simulink model "ESO_test"  (Simulink 8.8)
settings: Solver=ode45  StartTime=0.0  StopTime=10.0  RelTol=1e-3  EnableMultiTasking=on
values from neighbouring files (symbols this model uses):
  A = [-351.120003184 -5361.83522933 0 0 0 0 0 0 0 0 0 0 ... (196 elements, 14x14)]    [identified_modal.mat]    (also in identified_modal_250.mat = [-10.7295401852 -1238.51536589 0 0 0 0 1238.51536589 -10.729)
  Am = A    [ESO_performance_test.m]
  B = [573.623221602 72.4542684161 -691.638848987 228.937697811 -252.989182838 -22.7617436487 170.002545784 4.18017568557 -18.4488355601 113.905004057 -95.0717241213 -56.2996980805 ... (42 elements, 14x3)]    [identified_modal.mat]    (also in identified_modal_250.mat = [-1.29092394555 -1.97797965398 -0.850667801822 1.31545698651)
  Bm = B    [ESO_performance_test.m]
  C = [0.627446579032 0.0119792109415 0.587375916328 0.0249330272657 -0.39941806915 -0.0483765376125 0.228423611726 0.0697233755056 0.0235364777295 -0.0130974661322 0.147269800576 0.0117524583717 ... (28 elements, 2x14)]    [identified_modal.mat]    (also in identified_modal_250.mat = [-2.98376370972  6.90606082788  -5.3698593094  -1.7527268949)
  Cm = C    [ESO_performance_test.m]
  Cw = zeros(n_w,n_xw)    [ESO_design.m]    (also in ESO_performance_test.m)
  D = D(:,1:3)    [ESO_performance_test.m]    (also in identified_modal.mat = [-0.0335072369376  0.101109733478  0.0863325632373  -0.01405; identified_modal_250.mat = [-2.22661181806e-05  0.0283763020492  -0.000188131534199  0.)
  Dm = D    [ESO_performance_test.m]
  E = zeros(n_xw,n_h)    [ESO_design.m]    (also in ESO_performance_test.m)
  H = [33.6937621374 18.4906854499 -113.318027588 5.64627813379 9.51722897194 3.09854032404 -14.991856853 99.088587685 -7.37918928848 3.49318728719 21.2561682387 -20.6265244709 ... (14 elements, 14x1)]    [identified_modal.mat]    (also in identified_modal_250.mat = [0.0764124681014 0.0372004138976 0.178660840601 0.2484513591)
  Hm = H    [ESO_performance_test.m]
  L1 = L(1:n_x,:)    [ESO_performance_test.m]
  L2 = L(n_x+1:n_x+n_xw,:)    [ESO_performance_test.m]
  S = blkdiag(S,zeros(1,1))    [ESO_design.m]    (also in ESO_performance_test.m)
settings Model: Creator=Mehran  LastModifiedBy=ABLAH
settings OptimizationCC: ExpressionDepthLimit=2147483647
settings DebuggingCC: SolverPrmCheckMsg=warning

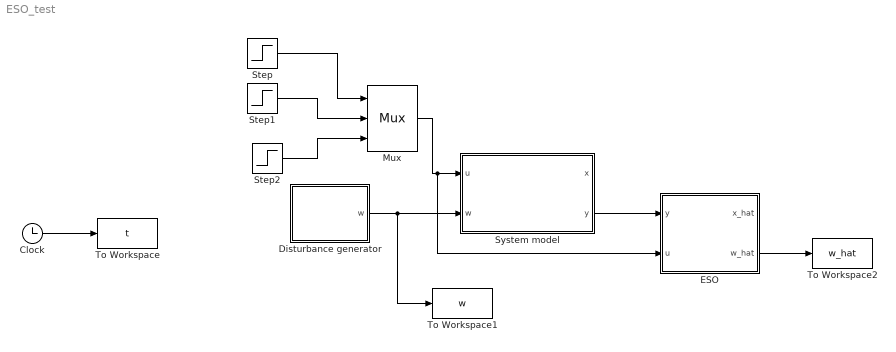
== system ESO_test ==
  Clock : Clock
  Disturbance generator : Subsystem
  ESO : Subsystem
  Mux : Mux  Inputs=3
  Step : Step  Time=0  After=0  SampleTime=0
  Step1 : Step  Time=0  After=0  SampleTime=0
  Step2 : Step  Time=0  After=0  SampleTime=0
  System model : Subsystem
  To Workspace : ToWorkspace  VariableName=t  SampleTime=-1
  To Workspace1 : ToWorkspace  VariableName=w  SampleTime=-1
  To Workspace2 : ToWorkspace  VariableName=w_hat  SampleTime=-1
  wires:
  Disturbance generator/1(w) -> System model/2(w), To Workspace1/1
  System model/2(y) -> ESO/1(y)
  Mux/1 -> System model/1(u), ESO/2(u)
  Step/1 -> Mux/1
  Step1/1 -> Mux/2
  Step2/1 -> Mux/3
  Clock/1 -> To Workspace/1
  ESO/2(w_hat) -> To Workspace2/1

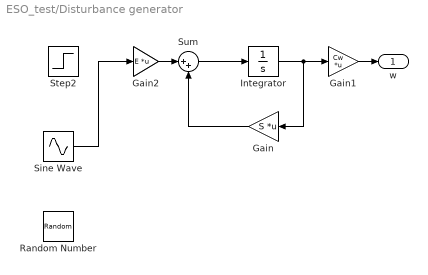
== system ESO_test/Disturbance generator ==
  Gain : Gain  Gain=S  Multiplication=Matrix(K*u)
  Gain1 : Gain  Gain=Cw  Multiplication=Matrix(K*u)
  Gain2 : Gain  Gain=E  Multiplication=Matrix(K*u)
  Integrator : Integrator  InitialCondition=0.1*[ones(12,1);0]
  Random Number : RandomNumber  SampleTime=0.1
  Sine Wave : Sin  Amplitude=3  Frequency=13.8  SampleTime=0
  Step2 : Step  Time=0  After=0  SampleTime=0
  Sum : Sum  Inputs=|++
  w : Outport
  wires:
  Integrator/1 -> Gain/1, Gain1/1
  Gain/1 -> Sum/2
  Sum/1 -> Integrator/1
  Gain1/1 -> w/1
  Gain2/1 -> Sum/1
  Sine Wave/1 -> Gain2/1

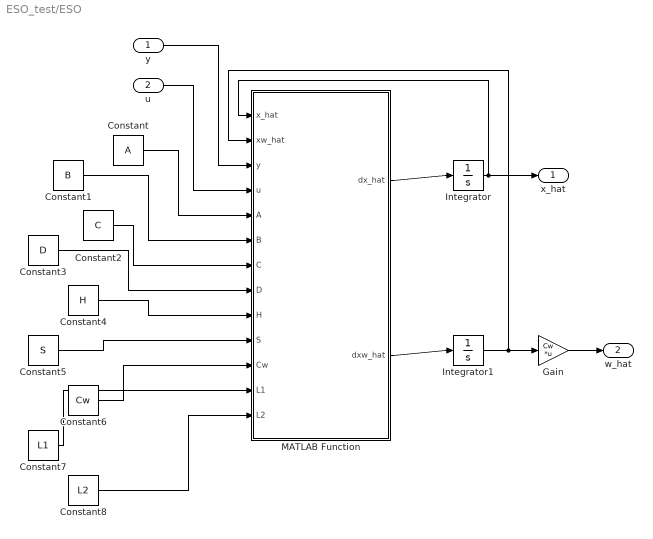
== system ESO_test/ESO ==
  y : Inport
  u : Inport  Port=2
  Constant : Constant  Value=A
  Constant1 : Constant  Value=B
  Constant2 : Constant  Value=C
  Constant3 : Constant  Value=D
  Constant4 : Constant  Value=H
  Constant5 : Constant  Value=S
  Constant6 : Constant  Value=Cw
  Constant7 : Constant  Value=L1
  Constant8 : Constant  Value=L2
  Gain : Gain  Gain=Cw  Multiplication=Matrix(K*u)
  Integrator : Integrator  InitialCondition=zeros(6,1)
  Integrator1 : Integrator  InitialCondition=zeros(13,1)
  MATLAB Function : MATLAB Function  TreatAsAtomicUnit=on
  x_hat : Outport
  w_hat : Outport  Port=2
  wires:
  MATLAB Function/1(dx_hat) -> Integrator/1
  MATLAB Function/2(dxw_hat) -> Integrator1/1
  Integrator/1 -> MATLAB Function/1(x_hat), x_hat/1
  Integrator1/1 -> MATLAB Function/2(xw_hat), Gain/1
  y/1 -> MATLAB Function/3(y)
  u/1 -> MATLAB Function/4(u)
  Constant/1 -> MATLAB Function/5(A)
  Constant1/1 -> MATLAB Function/6(B)
  Constant2/1 -> MATLAB Function/7(C)
  Constant3/1 -> MATLAB Function/8(D)
  Constant4/1 -> MATLAB Function/9(H)
  Constant5/1 -> MATLAB Function/10(S)
  Constant6/1 -> MATLAB Function/11(Cw)
  Constant7/1 -> MATLAB Function/12(L1)
  Constant8/1 -> MATLAB Function/13(L2)
  Gain/1 -> w_hat/1

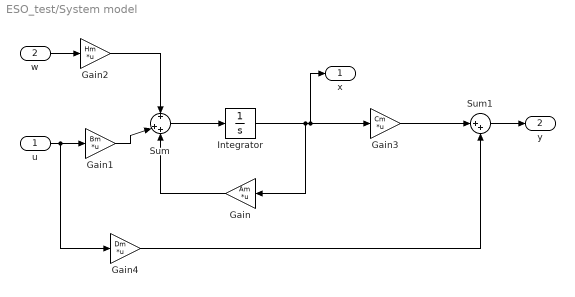
== system ESO_test/System model ==
  u : Inport
  w : Inport  Port=2
  Gain : Gain  Gain=Am  Multiplication=Matrix(K*u)
  Gain1 : Gain  Gain=Bm  Multiplication=Matrix(K*u)
  Gain2 : Gain  Gain=Hm  Multiplication=Matrix(K*u)
  Gain3 : Gain  Gain=Cm  Multiplication=Matrix(K*u)
  Gain4 : Gain  Gain=Dm  Multiplication=Matrix(K*u)
  Integrator : Integrator
  Sum : Sum  Inputs=+|++
  Sum1 : Sum  Inputs=|++
  x : Outport
  y : Outport  Port=2
  wires:
  Sum/1 -> Integrator/1
  Integrator/1 -> Gain3/1, x/1, Gain/1
  Gain/1 -> Sum/3
  Gain1/1 -> Sum/2
  u/1 -> Gain1/1, Gain4/1
  w/1 -> Gain2/1
  Gain2/1 -> Sum/1
  Gain3/1 -> Sum1/1
  Gain4/1 -> Sum1/2
  Sum1/1 -> y/1

== matlab function ESO/MATLAB Function ==
  data: x_hat input double; xw_hat input double; y input double; u input double; dx_hat output double; dxw_hat output double; A input double; B input double; C input double; D input double; H input double; S input double; Cw input double; L1 input double; L2 input double
function [dx_hat,dxw_hat] = ESO_dyn(x_hat,xw_hat,y,u,A,B,C,D,H,S,Cw,L1,L2)
dx_hat = zeros(6,1);
dxw_hat = zeros(13,1);
%% Gain function parameters
a = 0.7;
d = 0.1;
%% ESO DEs
dx_hat = A*x_hat+B*u+H*Cw'*xw_hat+L1*phi(y-C*x_hat-D*u,a,d);
dxw_hat = S*xw_hat+L2*phi(y-C*x_hat-D*u,a,d);
end
%Gain function
function y1 = phi(x1,a,d)
         y1 = zeros(2,1);
         y1(1) = x1(1) + 0.5*(a-1)*(abs(x1(1)+d)-abs(x1(1)-d));
         y1(2) = x1(2) + 0.5*(a-1)*(abs(x1(2)+d)-abs(x1(2)-d));
end
